simulink model "acceleration_from_encoder"  (R2022a)
settings: Solver=ode4  StartTime=0.0  StopTime=20/100  FixedStep=1e-3  RelTol=1e-3
undefined symbols (not defined in the file or in its folder): sensor, Ts_encoder
libraries: simulink x4, simulink_extras x1
settings Model: Creator=ahmad kourani  LastModifiedBy=ahmad kourani

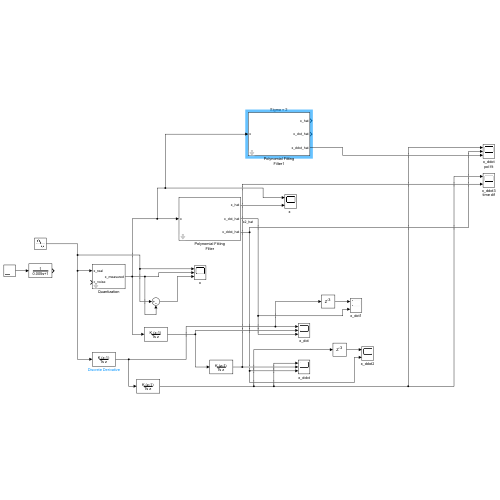
[thumbnail: Simulink's stored preview of the top-level diagram]
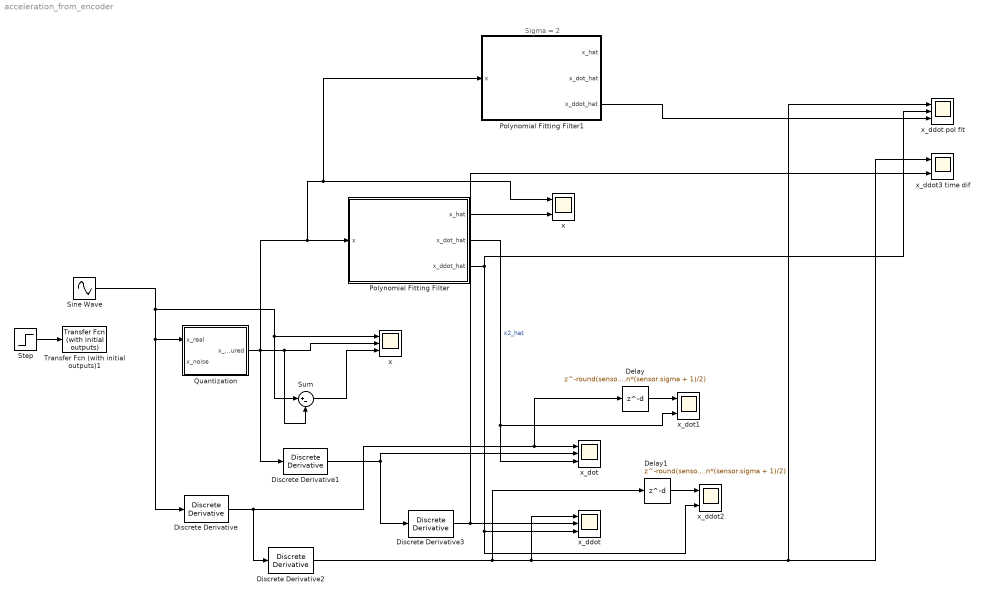
== system acceleration_from_encoder ==
  note: Sigma = 2
  Delay : Delay  DelayLength=round(sensor.n*(sensor.sigma + 1)/2)
  Delay1 : Delay  DelayLength=round(sensor.n*(sensor.sigma + 1)/2)
  Discrete Derivative{,1..3} (4 alike) : simulink/Discrete/Discrete Derivative  gainval=1.0  ICPrevScaledInput=0.0  OutMin=[]  OutMax=[]  OutDataType=fixdt(1, 16)  OutScaling=2^-10  DoSatur=off
  Polynomial Fitting Filter : Subsystem  mask{n=sensor.n, sigma=sensor.sigma, resolution=sensor.resolution, Ts_sensor=sensor.sample_time, Ts_estimation=sensor.estimation_time}
      mask prompts: n "number of sensor events to store:"; sigma "Skiped readings:"; resolution "sensor resolution:"; Ts_sensor "Sensor sample time (s):"; Ts_estimation "Estimation sample time (s):"
      mask init:
      | m = 2;
      |     t_k_star = [0:1/(n-1):1]'; %t_k/(n-1);
      |     A = [];
      |     for ii = m:-1:0
      |         A = [A t_k_star.^(ii)];
      |     end
  Polynomial Fitting Filter1 : Subsystem  mask{n=sensor.n, sigma=2, resolution=sensor.resolution, Ts_sensor=sensor.sample_time, Ts_estimation=sensor.estimation_time}
      mask prompts: n "number of sensor events to store:"; sigma "Skiped readings:"; resolution "sensor resolution:"; Ts_sensor "Sensor sample time (s):"; Ts_estimation "Estimation sample time (s):"
      mask init:
      | m = 2;
      |     t_k_star = [0:1/(n-1):1]'; %t_k/(n-1);
      |     A = [];
      |     for ii = m:-1:0
      |         A = [A t_k_star.^(ii)];
      |     end
  Quantization : Subsystem  SystemSampleTime=Ts_encoder  mask{FS=sensor.range, bits=sensor.bits_resolution}
      mask prompts: FS "Full Scale (range):"; bits "Number of bits:"
      mask init:
      | resolution = FS/2^bits;
  Sine Wave : Sin  Amplitude=10  Frequency=2*pi*10  SampleTime=0
  Step : Step  Time=0  After=10  SampleTime=0
  Sum : Sum  Inputs=|+-
  Transfer Fcn (with initial outputs)1 : simulink_extras/Additional Linear/Transfer Fcn (with initial outputs)  N=[1]  D=[5e-3 1]  Y0=0  U0=0
  x : Scope  NumInputPorts=3
  "x  " : Scope  NumInputPorts=2
  x_ddot : Scope  NumInputPorts=3
  x_ddot pol fit : Scope  NumInputPorts=3
  x_ddot2 : Scope  NumInputPorts=2
  x_ddot3 time dif : Scope  NumInputPorts=2
  x_dot : Scope  NumInputPorts=3
  x_dot1 : Scope  NumInputPorts=2
  wires:
  Step/1 -> Transfer Fcn (with initial outputs)1/1
  Quantization/1(x_measured) -> Polynomial Fitting Filter1/1(x), "x  "/1, Polynomial Fitting Filter/1(x), Discrete Derivative1/1, Sum/2, x/2
  Sine Wave/1 -> Discrete Derivative/1, Quantization/1(x_real), Sum/1, x/1
  Sum/1 -> x/3
  Discrete Derivative/1 -> Delay/1, x_dot/1, Discrete Derivative2/1
  Discrete Derivative1/1 -> Discrete Derivative3/1, x_dot/2
  Polynomial Fitting Filter/1(x_hat) -> "x  "/2
  Polynomial Fitting Filter/2(x_dot_hat) -> x_dot1/2, x_dot/3  "x2_hat"
  Discrete Derivative2/1 -> x_ddot3 time dif/1, x_ddot pol fit/1, x_ddot/1, Delay1/1
  Discrete Derivative3/1 -> x_ddot3 time dif/2, x_ddot/2
  Polynomial Fitting Filter/3(x_ddot_hat) -> x_ddot2/2, x_ddot/3, x_ddot pol fit/2
  Delay/1 -> x_dot1/1
  Delay1/1 -> x_ddot2/1
  Polynomial Fitting Filter1/3(x_ddot_hat) -> x_ddot pol fit/3

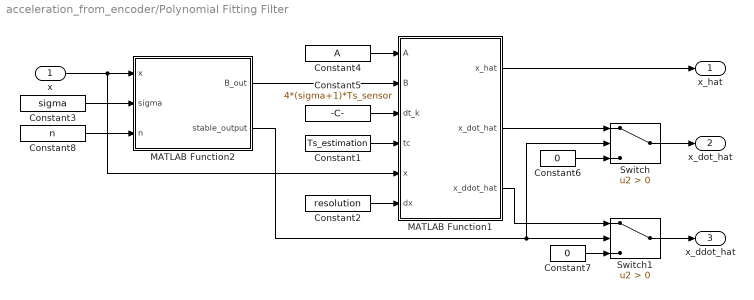
== system acceleration_from_encoder/Polynomial Fitting Filter ==
  x : Inport
  Constant1 : Constant  Value=Ts_estimation  OutDataTypeStr=double
  Constant2 : Constant  Value=resolution  OutDataTypeStr=double
  Constant3 : Constant  Value=sigma  OutDataTypeStr=double
  Constant4 : Constant  Value=A  OutDataTypeStr=double
  Constant5 : Constant  Value=4*(sigma+1)*Ts_sensor  OutDataTypeStr=double
  Constant6 : Constant  Value=0  OutDataTypeStr=double
  Constant7 : Constant  Value=0  OutDataTypeStr=double
  Constant8 : Constant  Value=n  OutDataTypeStr=double
  MATLAB Function1 : MATLAB Function  TreatAsAtomicUnit=on  SystemSampleTime=Ts_estimation
  MATLAB Function2 : MATLAB Function  TreatAsAtomicUnit=on  SystemSampleTime=Ts_sensor
  Switch : Switch  Criteria=u2 > Threshold  SaturateOnIntegerOverflow=off  InputSameDT=off
  Switch1 : Switch  Criteria=u2 > Threshold  SaturateOnIntegerOverflow=off  InputSameDT=off
  x_hat : Outport
  x_dot_hat : Outport  Port=2
  x_ddot_hat : Outport  Port=3
  wires:
  Constant3/1 -> MATLAB Function2/2(sigma)
  Constant2/1 -> MATLAB Function1/6(dx)
  x/1 -> MATLAB Function1/5(x), MATLAB Function2/1(x)
  Constant4/1 -> MATLAB Function1/1(A)
  Constant1/1 -> MATLAB Function1/4(tc)
  MATLAB Function1/1(x_hat) -> x_hat/1
  Constant5/1 -> MATLAB Function1/3(dt_k)
  Switch/1 -> x_dot_hat/1
  MATLAB Function1/2(x_dot_hat) -> Switch/1
  Constant6/1 -> Switch/3
  Switch1/1 -> x_ddot_hat/1
  MATLAB Function1/3(x_ddot_hat) -> Switch1/1
  Constant7/1 -> Switch1/3
  Constant8/1 -> MATLAB Function2/3(n)
  MATLAB Function2/1(B_out) -> MATLAB Function1/2(B)
  MATLAB Function2/2(stable_output) -> Switch1/2, Switch/2

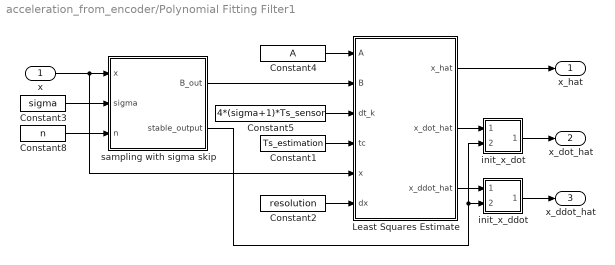
== system acceleration_from_encoder/Polynomial Fitting Filter1 ==
  x : Inport
  Constant1 : Constant  Value=Ts_estimation  OutDataTypeStr=double
  Constant2 : Constant  Value=resolution  OutDataTypeStr=double
  Constant3 : Constant  Value=sigma  OutDataTypeStr=double
  Constant4 : Constant  Value=A  OutDataTypeStr=double
  Constant5 : Constant  Value=4*(sigma+1)*Ts_sensor  OutDataTypeStr=double
  Constant8 : Constant  Value=n  OutDataTypeStr=double
  Least Squares Estimate : MATLAB Function  TreatAsAtomicUnit=on  SystemSampleTime=Ts_estimation
  init_x_ddot : Subsystem
  init_x_dot : Subsystem
  sampling with sigma skip : MATLAB Function  TreatAsAtomicUnit=on  SystemSampleTime=Ts_sensor
  x_hat : Outport
  x_dot_hat : Outport  Port=2
  x_ddot_hat : Outport  Port=3
  wires:
  sampling with sigma skip/2(stable_output) -> init_x_ddot/2(In2), init_x_dot/2(In2)
  sampling with sigma skip/1(B_out) -> Least Squares Estimate/2(B)
  Constant8/1 -> sampling with sigma skip/3(n)
  Constant5/1 -> Least Squares Estimate/3(dt_k)
  Least Squares Estimate/1(x_hat) -> x_hat/1
  Constant1/1 -> Least Squares Estimate/4(tc)
  Constant4/1 -> Least Squares Estimate/1(A)
  x/1 -> sampling with sigma skip/1(x), Least Squares Estimate/5(x)
  Constant2/1 -> Least Squares Estimate/6(dx)
  Constant3/1 -> sampling with sigma skip/2(sigma)
  Least Squares Estimate/2(x_dot_hat) -> init_x_dot/1(In1)
  init_x_dot/1(Out1) -> x_dot_hat/1
  Least Squares Estimate/3(x_ddot_hat) -> init_x_ddot/1(In1)
  init_x_ddot/1(Out1) -> x_ddot_hat/1

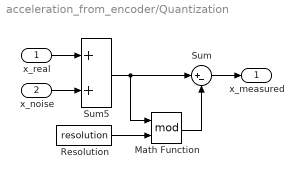
== system acceleration_from_encoder/Quantization ==
  x_real : Inport
  x_noise : Inport  Port=2
  Math Function : Math  Operator=mod  SignedPower=on
  "Resolution " : Constant  Value=resolution
  Sum : Sum  Inputs=|+-
  Sum5 : Sum  Inputs=2  InputSameDT=on  SaturateOnIntegerOverflow=on  OutDataTypeStr=Inherit: Same as first input
  x_measured : Outport  VectorParamsAs1DForOutWhenUnconnected=off
  wires:
  x_noise/1 -> Sum5/2
  Sum/1 -> x_measured/1
  x_real/1 -> Sum5/1
  Sum5/1 -> Sum/1, Math Function/1
  "Resolution "/1 -> Math Function/2
  Math Function/1 -> Sum/2

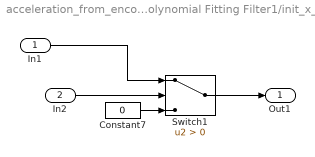
== system acceleration_from_encoder/Polynomial Fitting Filter1/init_x_ddot ==
  In1 : Inport
  In2 : Inport  Port=2
  Constant7 : Constant  Value=0  OutDataTypeStr=double
  Switch1 : Switch  Criteria=u2 > Threshold  SaturateOnIntegerOverflow=off  InputSameDT=off
  Out1 : Outport
  wires:
  Constant7/1 -> Switch1/3
  In2/1 -> Switch1/2
  In1/1 -> Switch1/1
  Switch1/1 -> Out1/1

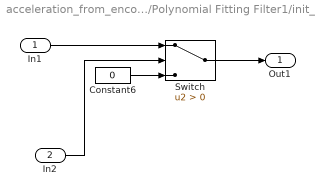
== system acceleration_from_encoder/Polynomial Fitting Filter1/init_x_dot ==
  In1 : Inport
  In2 : Inport  Port=2
  Constant6 : Constant  Value=0  OutDataTypeStr=double
  Switch : Switch  Criteria=u2 > Threshold  SaturateOnIntegerOverflow=off  InputSameDT=off
  Out1 : Outport
  wires:
  Constant6/1 -> Switch/3
  Switch/1 -> Out1/1
  In1/1 -> Switch/1
  In2/1 -> Switch/2

== matlab function acceleration_from_encoder/Polynomial Fitting Filter1/Least Squares Estimate ==
  data: A input; B input; dt_k input; tc input; x_hat output size=1; x input; dx input; x_dot_hat output size=1; x_ddot_hat output size=1
function [x_hat, x_dot_hat, x_ddot_hat] = ...
        LSE(A,B,dt_k,tc,x,dx) % P   ,A_out,B_out

P = zeros(3,1); % m = 2

P = (transpose(A)*A)\(transpose(A)*B);

x_hat = P'*[ (tc/dt_k)^2;(tc/dt_k)^1; 1];
x_dot_hat = P(1)*2*tc/dt_k^2 +  P(2)/dt_k;
x_ddot_hat =  2*P(1)/dt_k^2;

if abs(x_hat-x) > dx
    x_hat = x; 
end

== matlab function acceleration_from_encoder/Polynomial Fitting Filter1/sampling with sigma skip ==
  data: x input; B_out output; sigma input; stable_output output; n input
function [B_out,stable_output] = sampling(x,sigma,n)


% number of encoder events.
persistent B;
persistent skip;
persistent count_B;

n = 5;

if isempty(skip)
    skip = 0;
    B = zeros(n,1);
    count_B = 0;
end


if skip == 0
        B = [B(2:n); x];
        new = 1;
else
        new = 0;
end

%%
if new == 1 && count_B < n+1
    count_B = 1 + count_B;
end

if count_B == n+1
    stable_output = 1;
else
    stable_output = 0;
end

%%
skip = skip + 1;

if skip > sigma
    skip = 0;
end

B_out = B;

== matlab function acceleration_from_encoder/Polynomial Fitting Filter/MATLAB Function1 ==
  data: A input; B input; dt_k input; tc input; x_hat output size=1; x input; dx input; x_dot_hat output size=1; x_ddot_hat output size=1
function [x_hat, x_dot_hat, x_ddot_hat] = ...
        fcn(A,B,dt_k,tc,x,dx) % P   ,A_out,B_out

P = zeros(3,1); % m = 2

P = (transpose(A)*A)\(transpose(A)*B);

x_hat = P'*[ (tc/dt_k)^2;(tc/dt_k)^1; 1];
x_dot_hat = P(1)*2*tc/dt_k^2 +  P(2)/dt_k;
x_ddot_hat =  2*P(1)/dt_k^2;

if abs(x_hat-x) > dx
    x_hat = x; 
end

== matlab function acceleration_from_encoder/Polynomial Fitting Filter/MATLAB Function2 ==
  data: x input; B_out output; sigma input; stable_output output; n input
function [B_out,stable_output] = fcn(x,sigma,n)


% number of encoder events.
persistent B;
persistent skip;
persistent count_B;

n = 5;

if isempty(skip)
    skip = 0;
    B = zeros(n,1);
    count_B = 0;
end


if skip == 0
        B = [B(2:n); x];
        new = 1;
else
        new = 0;
end

%%
if new == 1 && count_B < n+1
    count_B = 1 + count_B;
end

if count_B == n+1
    stable_output = 1;
else
    stable_output = 0;
end

%%
skip = skip + 1;

if skip > sigma
    skip = 0;
end

B_out = B;
